simulink model "prob6"  (R2020b)
settings: Solver=FixedStepAuto  StartTime=0.0  StopTime=10.0  FixedStep=0.1  MaxStep=0.1  RelTol=1e-3
settings Model: Creator='Z'ome  LastModifiedBy='Z'ome
settings DataIOCC: SaveOutput=off  SaveTime=off

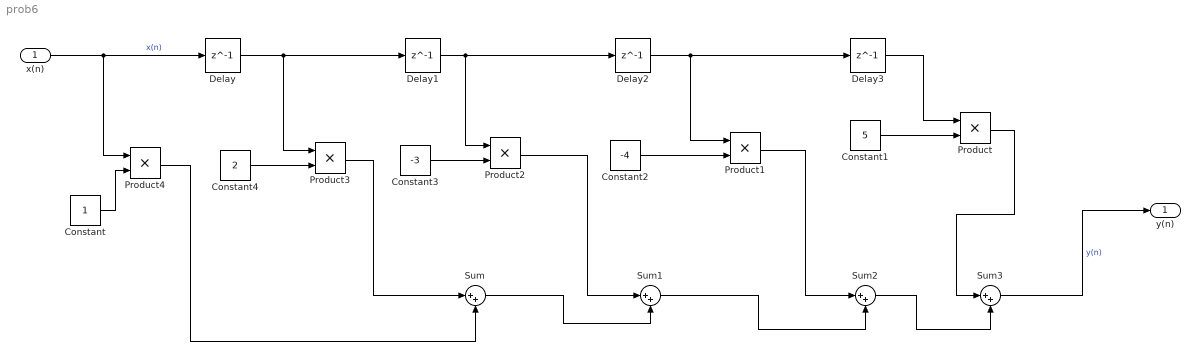
== system prob6 ==
  x(n) : Inport  OutDataTypeStr=double  PortDimensions=1  SampleTime=[0.10000000000000001,0]
  Constant : Constant
  Constant1 : Constant  Value=5
  Constant2 : Constant  Value=-4
  Constant3 : Constant  Value=-3
  Constant4 : Constant  Value=2
  Delay{,1..3} (4 alike) : Delay  DelayLength=1
  Product{,1..4} (5 alike) : Product
  Sum{,1..3} (4 alike) : Sum  Inputs=|++
  y(n) : Outport  OutDataTypeStr=double  PortDimensions=1  SampleTime=[0.10000000000000001,0]
  wires:
  Constant4/1 -> Product3/2
  Constant1/1 -> Product/2
  Sum/1 -> Sum1/2
  Delay/1 -> Product3/1, Delay1/1
  Constant/1 -> Product4/2
  Product4/1 -> Sum/2
  Constant3/1 -> Product2/2
  Sum1/1 -> Sum2/2
  Delay1/1 -> Product2/1, Delay2/1
  Product2/1 -> Sum1/1
  Constant2/1 -> Product1/2
  Sum2/1 -> Sum3/2
  Product/1 -> Sum3/1
  x(n)/1 -> Product4/1, Delay/1  "x(n)"
  Product1/1 -> Sum2/1
  Product3/1 -> Sum/1
  Delay3/1 -> Product/1
  Delay2/1 -> Product1/1, Delay3/1
  Sum3/1 -> y(n)/1  "y(n)"
